simulink library "findClosestPointOnPath"  (R2020a)
settings: Solver=VariableStepAuto  StartTime=0.0  StopTime=10.0  RelTol=1e-3
settings Model: Creator=Ayaz  LastModifiedBy=Ayaz

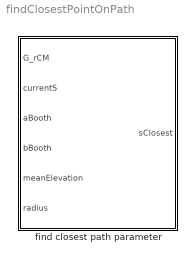
== system findClosestPointOnPath ==
  find closest path parameter : Subsystem

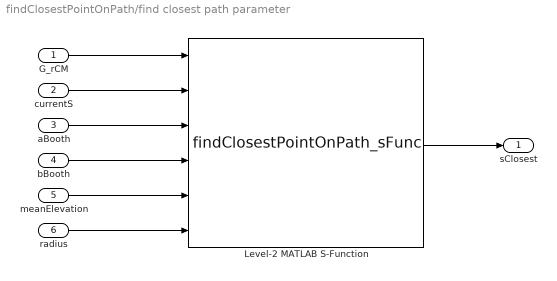
== system findClosestPointOnPath/find closest path parameter ==
  G_rCM : Inport
  currentS : Inport  Port=2
  aBooth : Inport  Port=3
  bBooth : Inport  Port=4
  meanElevation : Inport  Port=5
  radius : Inport  Port=6
  Level-2 MATLAB S-Function : M-S-Function  FunctionName=findClosestPointOnPath_sFunc
  sClosest : Outport
  wires:
  G_rCM/1 -> Level-2 MATLAB S-Function/1
  radius/1 -> Level-2 MATLAB S-Function/6
  meanElevation/1 -> Level-2 MATLAB S-Function/5
  bBooth/1 -> Level-2 MATLAB S-Function/4
  aBooth/1 -> Level-2 MATLAB S-Function/3
  currentS/1 -> Level-2 MATLAB S-Function/2
  Level-2 MATLAB S-Function/1 -> sClosest/1
